simulink model "sloworbcorr_ps_analog"  (Simulink 7.8)
settings: Solver=ode45  StartTime=0.0  StopTime=10.0  RelTol=1e-3
undefined symbols (not defined in the file or in its folder): simparam
settings Model: Creator=danielot  LastModifiedBy=danielot

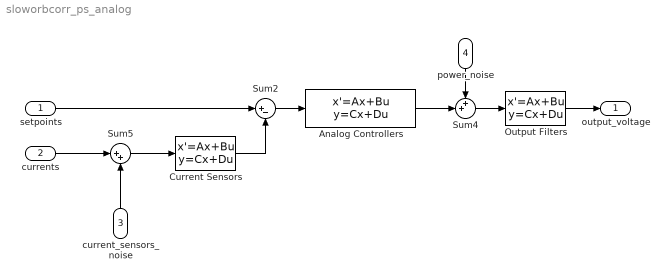
== system sloworbcorr_ps_analog ==
  setpoints : Inport
  currents : Inport  Port=2
  current_sensors_noise : Inport  Port=3
  power_noise : Inport  Port=4
  Analog Controllers : StateSpace  A=simparam.psctrl.a  B=simparam.psctrl.b  C=simparam.psctrl.c  D=simparam.psctrl.d
  Current Sensors : StateSpace  A=simparam.pssens.a  B=simparam.pssens.b  C=simparam.pssens.c  D=simparam.pssens.d
  Output Filters : StateSpace  A=simparam.psfilter.a  B=simparam.psfilter.b  C=simparam.psfilter.c  D=simparam.psfilter.d
  Sum2 : Sum  Inputs=|+-
  Sum4 : Sum  Inputs=++|
  Sum5 : Sum  Inputs=|++
  output_voltage : Outport
  wires:
  power_noise/1 -> Sum4/1
  current_sensors_noise/1 -> Sum5/2
  Sum5/1 -> Current Sensors/1
  currents/1 -> Sum5/1
  Output Filters/1 -> output_voltage/1
  Sum4/1 -> Output Filters/1
  Sum2/1 -> Analog Controllers/1
  Analog Controllers/1 -> Sum4/2
  setpoints/1 -> Sum2/1
  Current Sensors/1 -> Sum2/2
